simulink model "FOG_v5"  (R2023b)
settings: Solver=ode4  StartTime=0.0  StopTime=0.05  FixedStep=4.9999999999999998e-08  RelTol=1e-3
undefined symbols (not defined in the file): a_aa, b_aa, eta_conn, eta_dep, eta_K1, eta_pol, f_mod, I_dark_A, K1_detector_ratio, K1_launch_ratio, K_norm_digital, K_phase_to_deg, K_ref, K_sag, K_sagnac_power, noise_enable, noise_sample_scale, Omega_deg_s, P_source_W, phi0, q_e, ref_delay_total_s, Rf, Rpd, seed_dark, seed_johnson, seed_opamp_en, seed_opamp_i, seed_photo, sigma_dark_sample_A, sigma_johnson_sample_A, sigma_opamp_current_sample_A, sigma_opamp_voltage_sample_A, sos_d, tau, Ts_adc, Ts_noise, Vadc_max, Vadc_min, visibility, w_tia
settings Model: Creator=molik  LastModifiedBy=molik

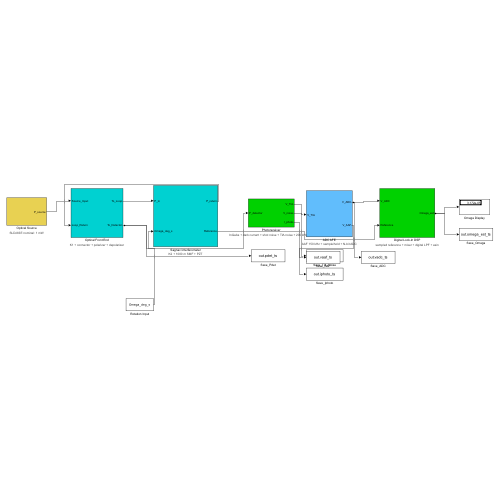
[thumbnail: Simulink's stored preview of the top-level diagram]
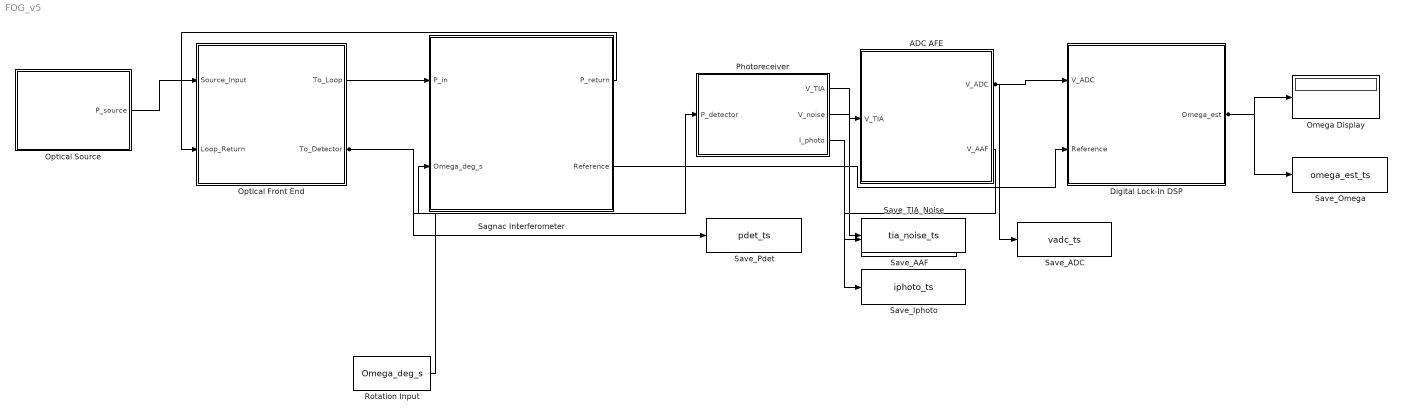
== system FOG_v5 ==
  ADC AFE : Subsystem
      settings: AttributesFormatString=AAF 150 kHz + sample/hold + N-bit ADC
  Digital Lock-In DSP : Subsystem
      settings: AttributesFormatString=sampled reference + mixer + digital LPF + asin
  Omega Display : Display
  Optical Front End : Subsystem
      settings: AttributesFormatString=K1 + connector + polarizer + depolarizer
  Optical Source : Subsystem
      settings: AttributesFormatString=SLD/ASE nominal: 1 mW
  Photoreceiver : Subsystem
      settings: AttributesFormatString=InGaAs + dark current + shot noise + TIA noise + 200 kHz BW
  Rotation Input : Constant  Value=Omega_deg_s
  Sagnac Interferometer : Subsystem
      settings: AttributesFormatString=K2 + 1000 m SMF + PZT
  Save_AAF : ToWorkspace  VariableName=vaaf_ts  SaveFormat=Timeseries  SampleTime=-1
  Save_ADC : ToWorkspace  VariableName=vadc_ts  SaveFormat=Timeseries  SampleTime=-1
  Save_Iphoto : ToWorkspace  VariableName=iphoto_ts  SaveFormat=Timeseries  SampleTime=-1
  Save_Omega : ToWorkspace  VariableName=omega_est_ts  SaveFormat=Timeseries  SampleTime=-1
  Save_Pdet : ToWorkspace  VariableName=pdet_ts  SaveFormat=Timeseries  SampleTime=-1
  Save_TIA_Noise : ToWorkspace  VariableName=tia_noise_ts  SaveFormat=Timeseries  SampleTime=-1
  wires:
  Optical Source/1(P_source) -> Optical Front End/1(Source_Input)
  Optical Front End/1(To_Loop) -> Sagnac Interferometer/1(P_in)
  Rotation Input/1 -> Sagnac Interferometer/2(Omega_deg_s)
  Sagnac Interferometer/1(P_return) -> Optical Front End/2(Loop_Return)
  Optical Front End/2(To_Detector) -> Save_Pdet/1, Photoreceiver/1(P_detector)
  Photoreceiver/2(V_noise) -> Save_TIA_Noise/1
  Photoreceiver/3(I_photo) -> Save_Iphoto/1
  Photoreceiver/1(V_TIA) -> ADC AFE/1(V_TIA)
  ADC AFE/1(V_ADC) -> Digital Lock-In DSP/1(V_ADC), Save_ADC/1
  Sagnac Interferometer/2(Reference) -> Digital Lock-In DSP/2(Reference)
  Digital Lock-In DSP/1(Omega_est) -> Omega Display/1, Save_Omega/1
  ADC AFE/2(V_AAF) -> Save_AAF/1

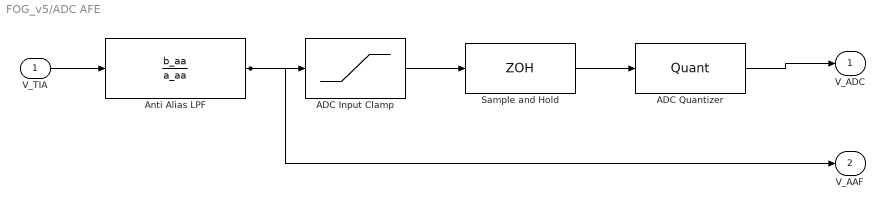
== system FOG_v5/ADC AFE ==
  V_TIA : Inport
  ADC Input Clamp : Saturate  UpperLimit=Vadc_max  LowerLimit=Vadc_min
  ADC Quantizer : Quantizer  QuantizationInterval=q_adc
  Anti Alias LPF : TransferFcn  Numerator=b_aa  Denominator=a_aa
  Sample and Hold : ZeroOrderHold  SampleTime=Ts_adc
  V_ADC : Outport
  V_AAF : Outport  Port=2
  wires:
  V_TIA/1 -> Anti Alias LPF/1
  Anti Alias LPF/1 -> ADC Input Clamp/1, V_AAF/1
  ADC Input Clamp/1 -> Sample and Hold/1
  Sample and Hold/1 -> ADC Quantizer/1
  ADC Quantizer/1 -> V_ADC/1

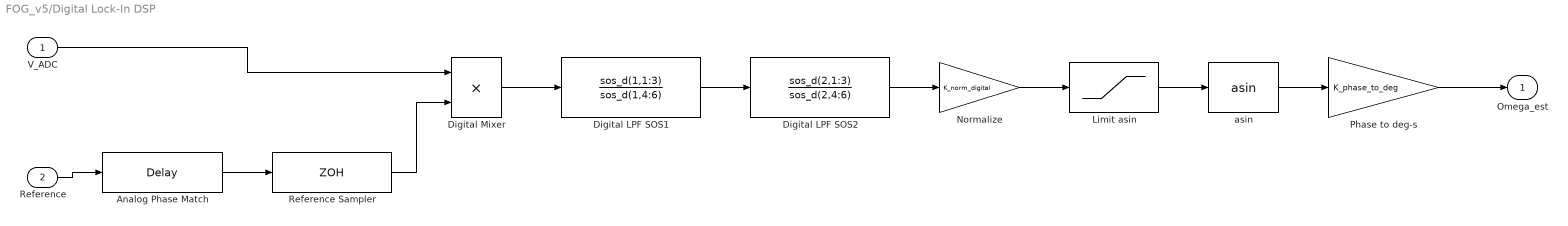
== system FOG_v5/Digital Lock-In DSP ==
  V_ADC : Inport
  Reference : Inport  Port=2
  Analog Phase Match : TransportDelay  DelayTime=ref_delay_total_s
  Digital LPF SOS1 : DiscreteTransferFcn  Numerator=sos_d(1,1:3)  Denominator=sos_d(1,4:6)  SampleTime=Ts_adc
  Digital LPF SOS2 : DiscreteTransferFcn  Numerator=sos_d(2,1:3)  Denominator=sos_d(2,4:6)  SampleTime=Ts_adc
  Digital Mixer : Product
  Limit asin : Saturate  UpperLimit=0.999999  LowerLimit=-0.999999
  Normalize : Gain  Gain=K_norm_digital
  Phase to deg-s : Gain  Gain=K_phase_to_deg
  Reference Sampler : ZeroOrderHold  SampleTime=Ts_adc
  asin : Trigonometry  Operator=asin
  Omega_est : Outport
  wires:
  V_ADC/1 -> Digital Mixer/1
  Reference/1 -> Analog Phase Match/1
  Analog Phase Match/1 -> Reference Sampler/1
  Reference Sampler/1 -> Digital Mixer/2
  Digital Mixer/1 -> Digital LPF SOS1/1
  Digital LPF SOS1/1 -> Digital LPF SOS2/1
  Digital LPF SOS2/1 -> Normalize/1
  Normalize/1 -> Limit asin/1
  Limit asin/1 -> asin/1
  asin/1 -> Phase to deg-s/1
  Phase to deg-s/1 -> Omega_est/1

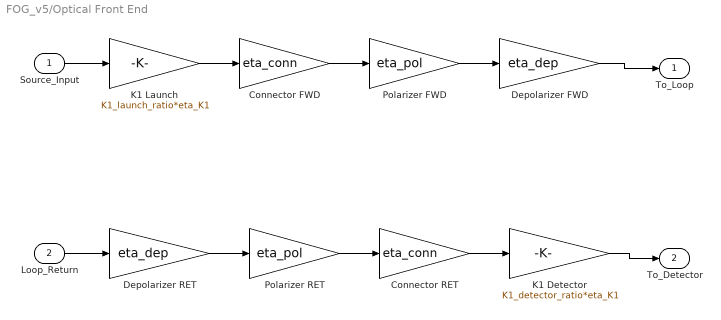
== system FOG_v5/Optical Front End ==
  Source_Input : Inport
  Loop_Return : Inport  Port=2
  Connector FWD : Gain  Gain=eta_conn
  Connector RET : Gain  Gain=eta_conn
  Depolarizer FWD : Gain  Gain=eta_dep
  Depolarizer RET : Gain  Gain=eta_dep
  K1 Detector : Gain  Gain=K1_detector_ratio*eta_K1
  K1 Launch : Gain  Gain=K1_launch_ratio*eta_K1
  Polarizer FWD : Gain  Gain=eta_pol
  Polarizer RET : Gain  Gain=eta_pol
  To_Loop : Outport
  To_Detector : Outport  Port=2
  wires:
  Source_Input/1 -> K1 Launch/1
  K1 Launch/1 -> Connector FWD/1
  Connector FWD/1 -> Polarizer FWD/1
  Polarizer FWD/1 -> Depolarizer FWD/1
  Depolarizer FWD/1 -> To_Loop/1
  Loop_Return/1 -> Depolarizer RET/1
  Depolarizer RET/1 -> Polarizer RET/1
  Polarizer RET/1 -> Connector RET/1
  Connector RET/1 -> K1 Detector/1
  K1 Detector/1 -> To_Detector/1

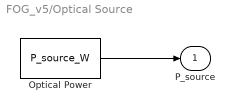
== system FOG_v5/Optical Source ==
  Optical Power : Constant  Value=P_source_W
  P_source : Outport
  wires:
  Optical Power/1 -> P_source/1

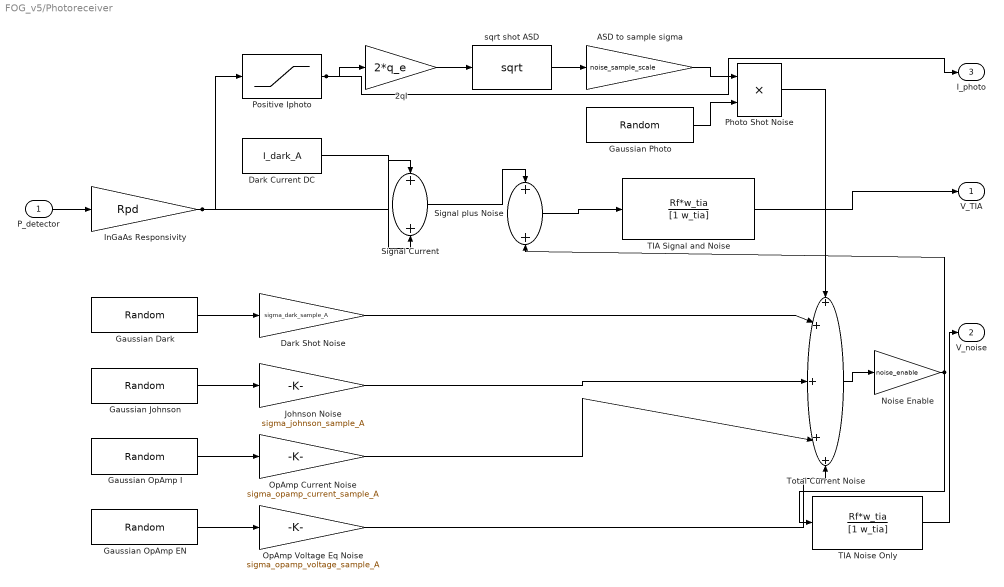
== system FOG_v5/Photoreceiver ==
  P_detector : Inport
  2qI : Gain  Gain=2*q_e
  ASD to sample sigma : Gain  Gain=noise_sample_scale
  Dark Current DC : Constant  Value=I_dark_A
  Dark Shot Noise : Gain  Gain=sigma_dark_sample_A
  Gaussian Dark : RandomNumber  Seed=seed_dark  SampleTime=Ts_noise
  Gaussian Johnson : RandomNumber  Seed=seed_johnson  SampleTime=Ts_noise
  Gaussian OpAmp EN : RandomNumber  Seed=seed_opamp_en  SampleTime=Ts_noise
  Gaussian OpAmp I : RandomNumber  Seed=seed_opamp_i  SampleTime=Ts_noise
  Gaussian Photo : RandomNumber  Seed=seed_photo  SampleTime=Ts_noise
  InGaAs Responsivity : Gain  Gain=Rpd
  Johnson Noise : Gain  Gain=sigma_johnson_sample_A
  Noise Enable : Gain  Gain=noise_enable
  OpAmp Current Noise : Gain  Gain=sigma_opamp_current_sample_A
  OpAmp Voltage Eq Noise : Gain  Gain=sigma_opamp_voltage_sample_A
  Photo Shot Noise : Product
  Positive Iphoto : Saturate  UpperLimit=inf  LowerLimit=0
  Signal Current : Sum
  Signal plus Noise : Sum
  TIA Noise Only : TransferFcn  Numerator=Rf*w_tia  Denominator=[1 w_tia]
  TIA Signal and Noise : TransferFcn  Numerator=Rf*w_tia  Denominator=[1 w_tia]
  Total Current Noise : Sum  Inputs=+++++
  sqrt shot ASD : Math  Operator=sqrt
  V_TIA : Outport
  V_noise : Outport  Port=2
  I_photo : Outport  Port=3
  wires:
  Gaussian Dark/1 -> Dark Shot Noise/1
  Gaussian Johnson/1 -> Johnson Noise/1
  Gaussian OpAmp I/1 -> OpAmp Current Noise/1
  Gaussian OpAmp EN/1 -> OpAmp Voltage Eq Noise/1
  P_detector/1 -> InGaAs Responsivity/1
  InGaAs Responsivity/1 -> Signal Current/1, Positive Iphoto/1
  Dark Current DC/1 -> Signal Current/2
  Signal Current/1 -> Signal plus Noise/1
  Noise Enable/1 -> Signal plus Noise/2, TIA Noise Only/1
  Signal plus Noise/1 -> TIA Signal and Noise/1
  TIA Signal and Noise/1 -> V_TIA/1
  Positive Iphoto/1 -> 2qI/1, I_photo/1
  2qI/1 -> sqrt shot ASD/1
  sqrt shot ASD/1 -> ASD to sample sigma/1
  ASD to sample sigma/1 -> Photo Shot Noise/1
  Gaussian Photo/1 -> Photo Shot Noise/2
  Photo Shot Noise/1 -> Total Current Noise/1
  Dark Shot Noise/1 -> Total Current Noise/2
  Johnson Noise/1 -> Total Current Noise/3
  OpAmp Current Noise/1 -> Total Current Noise/4
  OpAmp Voltage Eq Noise/1 -> Total Current Noise/5
  Total Current Noise/1 -> Noise Enable/1
  TIA Noise Only/1 -> V_noise/1

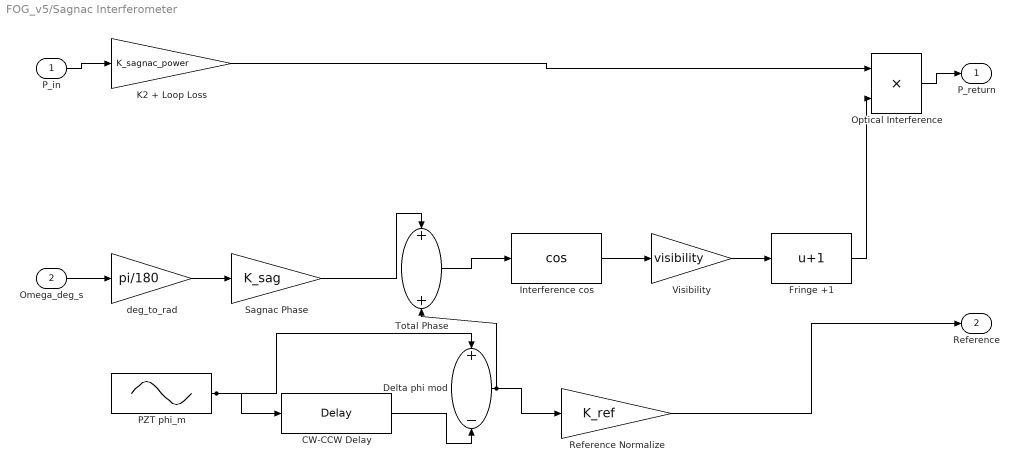
== system FOG_v5/Sagnac Interferometer ==
  P_in : Inport
  Omega_deg_s : Inport  Port=2
  CW-CCW Delay : TransportDelay  DelayTime=tau
  Delta phi mod : Sum  Inputs=+-
  Fringe +1 : Bias  Bias=1  SaturateOnIntegerOverflow=off
  Interference cos : Trigonometry  Operator=cos
  K2 + Loop Loss : Gain  Gain=K_sagnac_power
  Optical Interference : Product
  PZT phi_m : Sin  Amplitude=phi0  Frequency=2*pi*f_mod  SampleTime=0
  Reference Normalize : Gain  Gain=K_ref
  Sagnac Phase : Gain  Gain=K_sag
  Total Phase : Sum
  Visibility : Gain  Gain=visibility
  deg_to_rad : Gain  Gain=pi/180
  P_return : Outport
  Reference : Outport  Port=2
  wires:
  P_in/1 -> K2 + Loop Loss/1
  K2 + Loop Loss/1 -> Optical Interference/1
  Omega_deg_s/1 -> deg_to_rad/1
  deg_to_rad/1 -> Sagnac Phase/1
  Sagnac Phase/1 -> Total Phase/1
  PZT phi_m/1 -> Delta phi mod/1, CW-CCW Delay/1
  CW-CCW Delay/1 -> Delta phi mod/2
  Delta phi mod/1 -> Total Phase/2, Reference Normalize/1
  Total Phase/1 -> Interference cos/1
  Interference cos/1 -> Visibility/1
  Visibility/1 -> Fringe +1/1
  Fringe +1/1 -> Optical Interference/2
  Optical Interference/1 -> P_return/1
  Reference Normalize/1 -> Reference/1
